simulink model "jiaozhi_13"  (R2018a)
settings: Solver=VariableStepAuto  StartTime=0.0  StopTime=10.0  RelTol=1e-3
libraries: commrandsrc3 x2, commblkcod2 x2, commblkintrlv2 x1
settings Model: Creator=sdf  LastModifiedBy=sdf

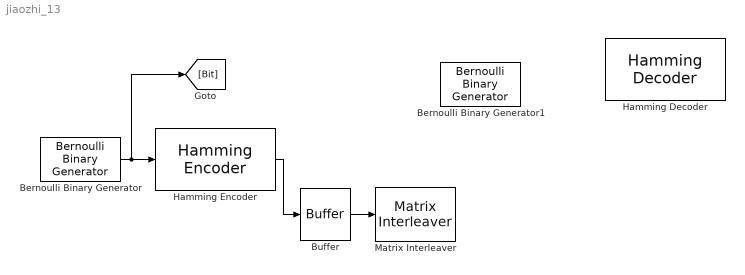
== system jiaozhi_13 ==
  Bernoulli Binary Generator : commrandsrc3/Bernoulli Binary Generator  ProbabilityOfZero=0.5  SeedSource=Parameter  Seed=61  SampleTime=1/110000  SamplesPerFrame=11  OutputDataType=double  SimulateUsing=Interpreted execution
  Bernoulli Binary Generator1 : commrandsrc3/Bernoulli Binary Generator  ProbabilityOfZero=0.001*ones(1,8)  SeedSource=Parameter  Seed=1234  SampleTime=1/150000  SamplesPerFrame=12  OutputDataType=double  SimulateUsing=Interpreted execution
  Buffer : Buffer  N=30*20  OutputFrames=off
  Hamming Decoder : commblkcod2/Hamming Decoder  n=15  k=11
      settings: SourceProductName=Communications System Toolbox  SourceProductBaseCode=CM
  Hamming Encoder : commblkcod2/Hamming Encoder  n=15  k=11
      settings: SourceProductName=Communications System Toolbox  SourceProductBaseCode=CM
  Matrix Interleaver : commblkintrlv2/Matrix Interleaver  Nrows=30  Ncols=20
      settings: SourceProductName=Communications System Toolbox  SourceProductBaseCode=CM
  wires:
  Bernoulli Binary Generator/1 -> [Bit], Hamming Encoder/1
  Hamming Encoder/1 -> Buffer/1
  Buffer/1 -> Matrix Interleaver/1
